simulink model "model"  (Simulink 7.4)
settings: Solver=ode5  StartTime=0.0  StopTime=inf  FixedStep=0.02  RelTol=1e-3
undefined symbols (not defined in the file or in its folder): Joystick, Standard_Devices
libraries: vrlib x6, rtwinlib x3
settings Model: Creator=Peter  LastModifiedBy=Peter  SimulationMode=external  CovHTMLOptions=-aTS=1 -bRG=1 -bTC=1 -hTR=0 -nFC=0 -scm=1 -bcm=1 -xEv=0  CovHtmlReporting=off  CovModelRefEnable=off
settings HardwareCC: ProdIntDivRoundTo=Zero  ProdEndianess=LittleEndian  ProdHWDeviceType=Generic->32-bit x86 compatible
settings RTWCC: SystemTargetFile=rtwin.tlc  TemplateMakefile=rtwin.tmf  Description=Real-Time Windows Target  ProcessScript=rtwin_make_rtw_hook  CustomInclude=emc  RTWCompilerOptimization=On
settings CodeAppCC: MaxIdLength=95
settings RTWinTargetCC: TargetLibSuffix=_rtwin.lib  TargetPreCompLibLocation=C:\Program Files\MATLAB\R2009b\toolbox\rtw\targets\rtwin\lib  TargetFunctionLibrary=ANSI_C  PortableWordSizes=off

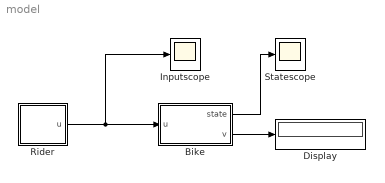
== system model ==
  Bike : Subsystem
  Display : Display
  Inputscope : Scope
  Rider : Subsystem
  Statescope : Scope
  wires:
  Bike/2(v) -> Display/1
  Bike/1(state) -> Statescope/1
  Rider/1(u) -> Bike/1(u), Inputscope/1

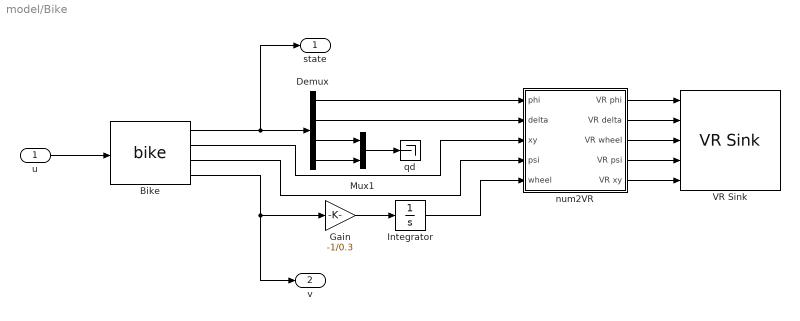
== system model/Bike ==
  u : Inport
  Bike : S-Function  InitFcn=try, set_param(gcb,'FunctionName','bike'), end  FunctionName=bike  SFunctionModules=bike_wrapper odefun_nonlinear rt_pow_snf  WizardData=DataTag0  EnableBusSupport=off  mask(S-Function Builder){}
      mask help: The S-Function Builder block creates a wrapper C-MEX S-function from your supplied C code with multiple input ports, output ports, and a variable number of scalar, vector, or matrix parameters. The input and output ports can propagate Simulink built-in data types, fixed-point datatypes, complex, frame, 1-D, and 2-D signals. This block also supports discrete and continuous states of type real. You can optionally have the block generate a TLC file to be used with Real-Time Workshop for code generation.
      mask init:
      | val = [[.9  0.75 0.75 1 1 .9 .9 1]',[1 1 0.75 0.75 .9 .9 1 .9]'];try , sys = get_param(gcb,'SfunBuilderFcnName');if isempty(sys), sys = get_param(gcb,'FunctionName'); end,catch, sys = get_param(gcb,'FunctionName'); end
      settings: CopyFcn=set_param(gcbh,'LinkStatus','none')  PreSaveFcn=try, set_param(gcb,'FunctionName','bike'), end  OpenFcn=sfunctionwizard(gcbh)
      mask Display: plot(val(:,1),val(:,2)),disp(sys)port_label('input',1,'u')port_label('output',1,'z')port_label('output',2,'xy')port_label('output',3,'psi')port_label('output',4,'v')
  Demux : Demux
  Gain : Gain  Gain=-1/0.3
  Integrator : Integrator
  Mux1 : Mux  Inputs=2
  VR Sink : vrlib/VR Sink  InstantiateOnLoad=on  SampleTime=0.02  ViewEnable=on  RemoteChange=off  RemoteView=off  FieldsWritten=phi.rotation.4.1.double#delta.rotation.4.1.double#rw_help.rotation.4.1.double#psi_grid.rotation.4.1.double#grid.translation.3.1.double  WorldFileName=bicycle.WRL  AutoView=off  VideoDimensions=[]
  num2VR : Subsystem
  qd : Terminator
  state : Outport
  v : Outport  Port=2  OutDataType=fixdt(1, 16)  OutScaling=2^0
  wires:
  u/1 -> Bike/1
  Demux/1 -> num2VR/1(phi)
  Bike/1 -> Demux/1, state/1
  Demux/2 -> num2VR/2(delta)
  Demux/3 -> Mux1/1
  Demux/4 -> Mux1/2
  Mux1/1 -> qd/1
  Gain/1 -> Integrator/1
  Integrator/1 -> num2VR/5(wheel)
  Bike/3 -> num2VR/4(psi)
  Bike/4 -> Gain/1, v/1
  Bike/2 -> num2VR/3(xy)
  num2VR/1(VR phi) -> VR Sink/1
  num2VR/2(VR delta) -> VR Sink/2
  num2VR/3(VR wheel) -> VR Sink/3
  num2VR/4(VR psi) -> VR Sink/4
  num2VR/5(VR xy) -> VR Sink/5

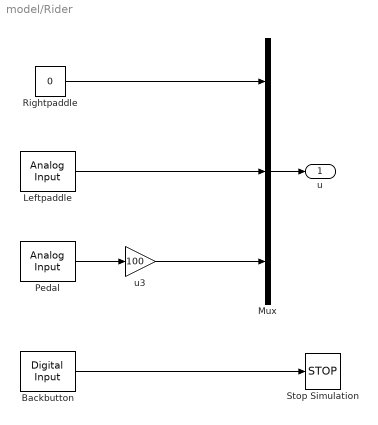
== system model/Rider ==
  Backbutton : rtwinlib/Digital Input  SampleTime=0.02  DrvName=Standard_Devices/Joystick  DrvAddress=1  DrvOptions=zeros(1,0)  Channels=7  BitMode=1  DataType=1
      settings: AttributesFormatString=Standard Devices\nJoystick [1h]
  Leftpaddle : rtwinlib/Analog Input  SampleTime=0.02  DrvName=Standard_Devices/Joystick  DrvAddress=1  DrvOptions=zeros(1,0)  Channels=1  RangeMode=1  VoltRange=1  DataType=1
      settings: AttributesFormatString=Standard Devices\nJoystick [1h]
  Mux : Mux  Inputs=3
  Pedal : rtwinlib/Analog Input  SampleTime=0.02  DrvName=Standard_Devices/Joystick  DrvAddress=1  DrvOptions=zeros(1,0)  Channels=3  RangeMode=1  VoltRange=1  DataType=1
      settings: AttributesFormatString=Standard Devices\nJoystick [1h]
  Rightpaddle : Constant  Value=0  OutDataType=fixdt(1, 16)  OutScaling=2^0
  Stop Simulation : Stop
  u3 : Gain  Gain=100
  u : Outport
  wires:
  Mux/1 -> u/1
  Pedal/1 -> u3/1
  u3/1 -> Mux/3
  Rightpaddle/1 -> Mux/1
  Backbutton/1 -> Stop Simulation/1
  Leftpaddle/1 -> Mux/2

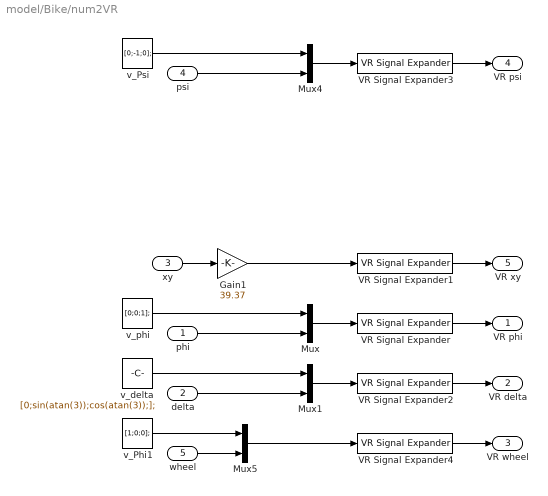
== system model/Bike/num2VR ==
  phi : Inport
  delta : Inport  Port=2
  xy : Inport  Port=3
  psi : Inport  Port=4
  wheel : Inport  Port=5
  Gain1 : Gain  Gain=39.37
  Mux{,1,4..5} (4 alike) : Mux  Inputs=2
  VR Signal Expander{,2..4} (4 alike) : vrlib/VR Signal Expander  SystemSampleTime=-1  outwidth=4  outidx=[1 2 3 4]
  VR Signal Expander1 : vrlib/VR Signal Expander  SystemSampleTime=-1  outwidth=3  outidx=[3 1]
  v_Phi1 : Constant  Value=[1;0;0];
  v_Psi : Constant  Value=[0;-1;0];
  v_delta : Constant  Value=[0;sin(atan(3));cos(atan(3));];
  v_phi : Constant  Value=[0;0;1];
  VR phi : Outport
  VR delta : Outport  Port=2
  VR wheel : Outport  Port=3
  VR psi : Outport  Port=4
  VR xy : Outport  Port=5
  wires:
  psi/1 -> Mux4/2
  v_Psi/1 -> Mux4/1
  Mux4/1 -> VR Signal Expander3/1
  VR Signal Expander3/1 -> VR psi/1
  VR Signal Expander1/1 -> VR xy/1
  v_phi/1 -> Mux/1
  Mux/1 -> VR Signal Expander/1
  phi/1 -> Mux/2
  VR Signal Expander/1 -> VR phi/1
  Mux1/1 -> VR Signal Expander2/1
  v_delta/1 -> Mux1/1
  delta/1 -> Mux1/2
  VR Signal Expander2/1 -> VR delta/1
  v_Phi1/1 -> Mux5/1
  Mux5/1 -> VR Signal Expander4/1
  wheel/1 -> Mux5/2
  VR Signal Expander4/1 -> VR wheel/1
  xy/1 -> Gain1/1
  Gain1/1 -> VR Signal Expander1/1
